simulink model "first_b"  (R2017a)
settings: Solver=VariableStepAuto  StartTime=0.0  StopTime=10.0  RelTol=1e-3
undefined symbols (not defined in the file): C1, C2, L1, R1, R2
settings Model: Creator=user  LastModifiedBy=user

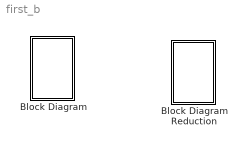
== system first_b ==
  Block Diagram : Subsystem
  Block Diagram Reduction : Subsystem

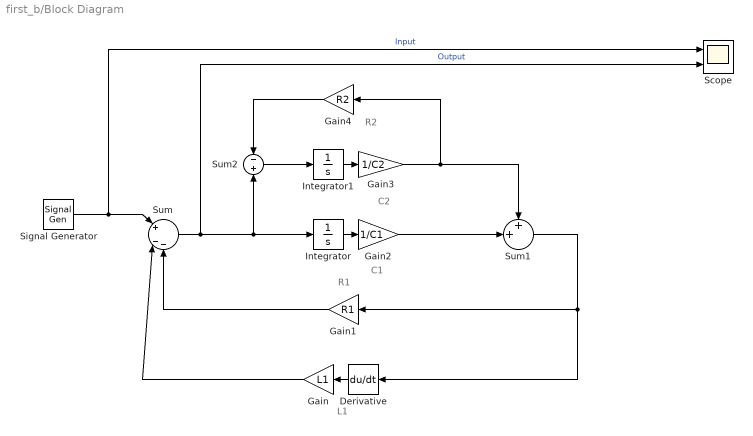
== system first_b/Block Diagram ==
  note: R2
  note: C2
  note: C1
  note: L1
  note: R1
  Derivative : Derivative  CoefficientInTFapproximation=0
  Gain : Gain  Gain=L1
  Gain1 : Gain  Gain=R1
  Gain2 : Gain  Gain=1/C1
  Gain3 : Gain  Gain=1/C2
  Gain4 : Gain  Gain=R2
  Integrator : Integrator
  Integrator1 : Integrator
  Scope : Scope  NumInputPorts=2
  Signal Generator : SignalGenerator  Units=rad/sec
  Sum : Sum  Inputs=|+|--
  Sum1 : Sum  Inputs=++|
  Sum2 : Sum  Inputs=-+
  wires:
  Gain1/1 -> Sum/3
  Derivative/1 -> Gain/1
  Gain/1 -> Sum/2
  Sum/1 -> Scope/2, Sum2/2, Integrator/1  "Output"
  Integrator/1 -> Gain2/1
  Gain2/1 -> Sum1/2
  Sum2/1 -> Integrator1/1
  Integrator1/1 -> Gain3/1
  Gain3/1 -> Gain4/1, Sum1/1
  Gain4/1 -> Sum2/1
  Sum1/1 -> Derivative/1, Gain1/1
  Signal Generator/1 -> Scope/1, Sum/1  "Input"

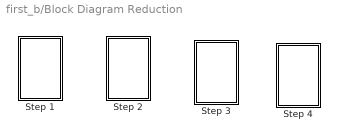
== system first_b/Block Diagram Reduction ==
  Step 1 : Subsystem
  Step 2 : Subsystem
  Step 3 : Subsystem
  Step 4 : Subsystem

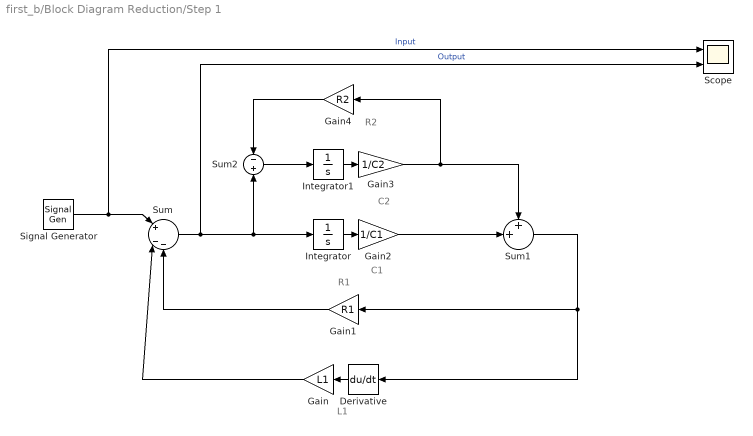
== system first_b/Block Diagram Reduction/Step 1 ==
  note: R1
  note: L1
  note: C1
  note: C2
  note: R2
  Derivative : Derivative  CoefficientInTFapproximation=0
  Gain : Gain  Gain=L1
  Gain1 : Gain  Gain=R1
  Gain2 : Gain  Gain=1/C1
  Gain3 : Gain  Gain=1/C2
  Gain4 : Gain  Gain=R2
  Integrator : Integrator
  Integrator1 : Integrator
  Scope : Scope  NumInputPorts=2
  Signal Generator : SignalGenerator  Units=rad/sec
  Sum : Sum  Inputs=|+|--
  Sum1 : Sum  Inputs=++|
  Sum2 : Sum  Inputs=-+
  wires:
  Gain1/1 -> Sum/3
  Gain2/1 -> Sum1/2
  Sum2/1 -> Integrator1/1
  Integrator1/1 -> Gain3/1
  Gain3/1 -> Gain4/1, Sum1/1
  Gain4/1 -> Sum2/1
  Sum1/1 -> Derivative/1, Gain1/1
  Signal Generator/1 -> Scope/1, Sum/1  "Input"
  Sum/1 -> Scope/2, Sum2/2, Integrator/1  "Output"
  Integrator/1 -> Gain2/1
  Gain/1 -> Sum/2
  Derivative/1 -> Gain/1

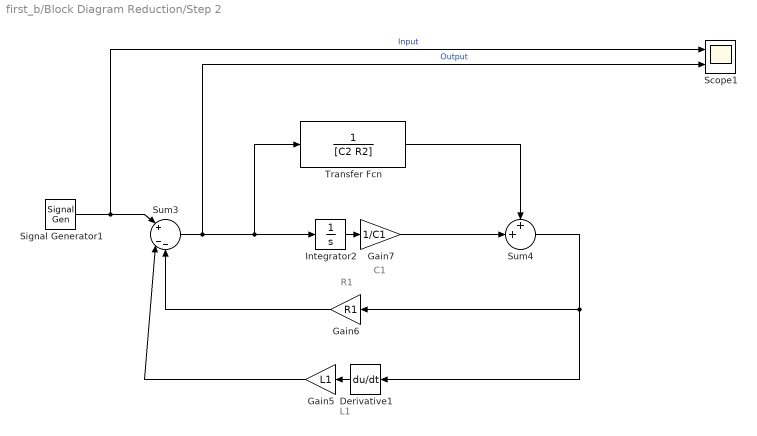
== system first_b/Block Diagram Reduction/Step 2 ==
  note: C1
  note: R1
  note: L1
  Derivative1 : Derivative  CoefficientInTFapproximation=0
  Gain5 : Gain  Gain=L1
  Gain6 : Gain  Gain=R1
  Gain7 : Gain  Gain=1/C1
  Integrator2 : Integrator
  Scope1 : Scope  NumInputPorts=2
  Signal Generator1 : SignalGenerator  Units=rad/sec
  Sum3 : Sum  Inputs=|+|--
  Sum4 : Sum  Inputs=++|
  Transfer Fcn : TransferFcn  Denominator=[C2 R2]
  wires:
  Sum3/1 -> Scope1/2, Transfer Fcn/1, Integrator2/1  "Output"
  Gain6/1 -> Sum3/3
  Transfer Fcn/1 -> Sum4/1
  Gain5/1 -> Sum3/2
  Sum4/1 -> Derivative1/1, Gain6/1
  Derivative1/1 -> Gain5/1
  Integrator2/1 -> Gain7/1
  Signal Generator1/1 -> Scope1/1, Sum3/1  "Input"
  Gain7/1 -> Sum4/2

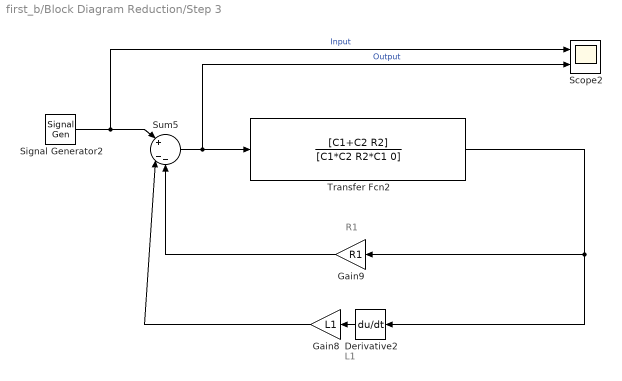
== system first_b/Block Diagram Reduction/Step 3 ==
  note: L1
  note: R1
  Derivative2 : Derivative  CoefficientInTFapproximation=0
  Gain8 : Gain  Gain=L1
  Gain9 : Gain  Gain=R1
  Scope2 : Scope  NumInputPorts=2
  Signal Generator2 : SignalGenerator  Units=rad/sec
  Sum5 : Sum  Inputs=|+|--
  Transfer Fcn2 : TransferFcn  Numerator=[C1+C2 R2]  Denominator=[C1*C2 R2*C1 0]
  wires:
  Derivative2/1 -> Gain8/1
  Signal Generator2/1 -> Scope2/1, Sum5/1  "Input"
  Gain9/1 -> Sum5/3
  Transfer Fcn2/1 -> Derivative2/1, Gain9/1
  Sum5/1 -> Scope2/2, Transfer Fcn2/1  "Output"
  Gain8/1 -> Sum5/2

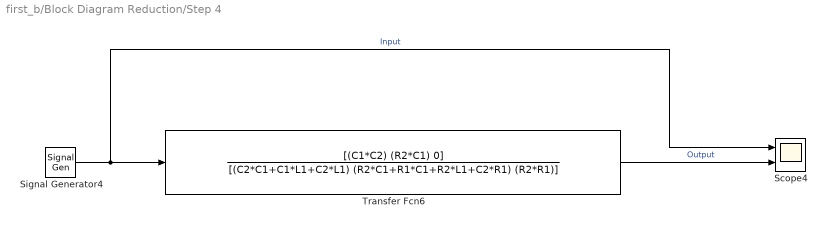
== system first_b/Block Diagram Reduction/Step 4 ==
  Scope4 : Scope  NumInputPorts=2
  Signal Generator4 : SignalGenerator  Units=rad/sec
  Transfer Fcn6 : TransferFcn  Numerator=[(C1*C2) (R2*C1) 0]  Denominator=[(C2*C1+C1*L1+C2*L1) (R2*C1+R1*C1+R2*L1+C2*R1) (R2*R1)]
  wires:
  Transfer Fcn6/1 -> Scope4/2  "Output"
  Signal Generator4/1 -> Scope4/1, Transfer Fcn6/1  "Input"
